simulink model "PTTransmCU"  (Simulink 10.3)
settings: Solver=ode45  StartTime=0.0  StopTime=inf  RelTol=1e-3  EnableMultiTasking=on
libraries: simulink x2, CarMaker4SL x1
(part 5 of 5)

== system PTTransmCU/CarMaker/IPG Vehicle/PowerTrain/TCU Example/TCU GearboxOut/CreateBus TCU GearboxOut0 ==
  In : Inport
  BusCreator : BusCreator  Inputs=7
  Demux : Demux  Outputs=7
      settings: DisplayOption=none
  Out : Outport  VectorParamsAs1DForOutWhenUnconnected=off
  wires:
  Demux/7 -> BusCreator/7  "TCU GearboxOut0 Clutch_dis Pos"
  Demux/6 -> BusCreator/6  "TCU GearboxOut0 Clutch Pos"
  Demux/5 -> BusCreator/5  "TCU GearboxOut0 i_trg"
  Demux/4 -> BusCreator/4  "TCU GearboxOut0 Trq_DriveSrc_trg"
  Demux/3 -> BusCreator/3  "TCU GearboxOut0 set_ParkBrake"
  Demux/2 -> BusCreator/2  "TCU GearboxOut0 GearNoTrg_dis"
  Demux/1 -> BusCreator/1  "TCU GearboxOut0 GearNoTrg"
  BusCreator/1 -> Out/1
  In/1 -> Demux/1

== system PTTransmCU/CarMaker/IPG Vehicle/PowerTrain/TCU Example/TCU GearboxOut/CreateBus TCU GearboxOut1 ==
  In : Inport
  BusCreator : BusCreator  Inputs=7
  Demux : Demux  Outputs=7
      settings: DisplayOption=none
  Out : Outport  VectorParamsAs1DForOutWhenUnconnected=off
  wires:
  Demux/7 -> BusCreator/7  "TCU GearboxOut1 Clutch_dis Pos"
  Demux/6 -> BusCreator/6  "TCU GearboxOut1 Clutch Pos"
  Demux/5 -> BusCreator/5  "TCU GearboxOut1 i_trg"
  Demux/4 -> BusCreator/4  "TCU GearboxOut1 Trq_DriveSrc_trg"
  Demux/3 -> BusCreator/3  "TCU GearboxOut1 set_ParkBrake"
  Demux/2 -> BusCreator/2  "TCU GearboxOut1 GearNoTrg_dis"
  Demux/1 -> BusCreator/1  "TCU GearboxOut1 GearNoTrg"
  BusCreator/1 -> Out/1
  In/1 -> Demux/1

== system PTTransmCU/CarMaker/IPG Vehicle/PowerTrain/TCU Example/TCU GearboxOut/CreateBus TCU GearboxOut10 ==
  In : Inport
  BusCreator : BusCreator  Inputs=7
  Demux : Demux  Outputs=7
      settings: DisplayOption=none
  Out : Outport  VectorParamsAs1DForOutWhenUnconnected=off
  wires:
  Demux/7 -> BusCreator/7  "TCU GearboxOut10 Clutch_dis Pos"
  Demux/6 -> BusCreator/6  "TCU GearboxOut10 Clutch Pos"
  Demux/5 -> BusCreator/5  "TCU GearboxOut10 i_trg"
  Demux/4 -> BusCreator/4  "TCU GearboxOut10 Trq_DriveSrc_trg"
  Demux/3 -> BusCreator/3  "TCU GearboxOut10 set_ParkBrake"
  Demux/2 -> BusCreator/2  "TCU GearboxOut10 GearNoTrg_dis"
  Demux/1 -> BusCreator/1  "TCU GearboxOut10 GearNoTrg"
  BusCreator/1 -> Out/1
  In/1 -> Demux/1

== system PTTransmCU/CarMaker/IPG Vehicle/PowerTrain/TCU Example/TCU GearboxOut/CreateBus TCU GearboxOut11 ==
  In : Inport
  BusCreator : BusCreator  Inputs=7
  Demux : Demux  Outputs=7
      settings: DisplayOption=none
  Out : Outport  VectorParamsAs1DForOutWhenUnconnected=off
  wires:
  Demux/7 -> BusCreator/7  "TCU GearboxOut11 Clutch_dis Pos"
  Demux/6 -> BusCreator/6  "TCU GearboxOut11 Clutch Pos"
  Demux/5 -> BusCreator/5  "TCU GearboxOut11 i_trg"
  Demux/4 -> BusCreator/4  "TCU GearboxOut11 Trq_DriveSrc_trg"
  Demux/3 -> BusCreator/3  "TCU GearboxOut11 set_ParkBrake"
  Demux/2 -> BusCreator/2  "TCU GearboxOut11 GearNoTrg_dis"
  Demux/1 -> BusCreator/1  "TCU GearboxOut11 GearNoTrg"
  BusCreator/1 -> Out/1
  In/1 -> Demux/1

== system PTTransmCU/CarMaker/IPG Vehicle/PowerTrain/TCU Example/TCU GearboxOut/CreateBus TCU GearboxOut2 ==
  In : Inport
  BusCreator : BusCreator  Inputs=7
  Demux : Demux  Outputs=7
      settings: DisplayOption=none
  Out : Outport  VectorParamsAs1DForOutWhenUnconnected=off
  wires:
  Demux/7 -> BusCreator/7  "TCU GearboxOut2 Clutch_dis Pos"
  Demux/6 -> BusCreator/6  "TCU GearboxOut2 Clutch Pos"
  Demux/5 -> BusCreator/5  "TCU GearboxOut2 i_trg"
  Demux/4 -> BusCreator/4  "TCU GearboxOut2 Trq_DriveSrc_trg"
  Demux/3 -> BusCreator/3  "TCU GearboxOut2 set_ParkBrake"
  Demux/2 -> BusCreator/2  "TCU GearboxOut2 GearNoTrg_dis"
  Demux/1 -> BusCreator/1  "TCU GearboxOut2 GearNoTrg"
  BusCreator/1 -> Out/1
  In/1 -> Demux/1

== system PTTransmCU/CarMaker/IPG Vehicle/PowerTrain/TCU Example/TCU GearboxOut/CreateBus TCU GearboxOut3 ==
  In : Inport
  BusCreator : BusCreator  Inputs=7
  Demux : Demux  Outputs=7
      settings: DisplayOption=none
  Out : Outport  VectorParamsAs1DForOutWhenUnconnected=off
  wires:
  Demux/7 -> BusCreator/7  "TCU GearboxOut3 Clutch_dis Pos"
  Demux/6 -> BusCreator/6  "TCU GearboxOut3 Clutch Pos"
  Demux/5 -> BusCreator/5  "TCU GearboxOut3 i_trg"
  Demux/4 -> BusCreator/4  "TCU GearboxOut3 Trq_DriveSrc_trg"
  Demux/3 -> BusCreator/3  "TCU GearboxOut3 set_ParkBrake"
  Demux/2 -> BusCreator/2  "TCU GearboxOut3 GearNoTrg_dis"
  Demux/1 -> BusCreator/1  "TCU GearboxOut3 GearNoTrg"
  BusCreator/1 -> Out/1
  In/1 -> Demux/1

== system PTTransmCU/CarMaker/IPG Vehicle/PowerTrain/TCU Example/TCU GearboxOut/CreateBus TCU GearboxOut4 ==
  In : Inport
  BusCreator : BusCreator  Inputs=7
  Demux : Demux  Outputs=7
      settings: DisplayOption=none
  Out : Outport  VectorParamsAs1DForOutWhenUnconnected=off
  wires:
  Demux/7 -> BusCreator/7  "TCU GearboxOut4 Clutch_dis Pos"
  Demux/6 -> BusCreator/6  "TCU GearboxOut4 Clutch Pos"
  Demux/5 -> BusCreator/5  "TCU GearboxOut4 i_trg"
  Demux/4 -> BusCreator/4  "TCU GearboxOut4 Trq_DriveSrc_trg"
  Demux/3 -> BusCreator/3  "TCU GearboxOut4 set_ParkBrake"
  Demux/2 -> BusCreator/2  "TCU GearboxOut4 GearNoTrg_dis"
  Demux/1 -> BusCreator/1  "TCU GearboxOut4 GearNoTrg"
  BusCreator/1 -> Out/1
  In/1 -> Demux/1

== system PTTransmCU/CarMaker/IPG Vehicle/PowerTrain/TCU Example/TCU GearboxOut/CreateBus TCU GearboxOut5 ==
  In : Inport
  BusCreator : BusCreator  Inputs=7
  Demux : Demux  Outputs=7
      settings: DisplayOption=none
  Out : Outport  VectorParamsAs1DForOutWhenUnconnected=off
  wires:
  Demux/7 -> BusCreator/7  "TCU GearboxOut5 Clutch_dis Pos"
  Demux/6 -> BusCreator/6  "TCU GearboxOut5 Clutch Pos"
  Demux/5 -> BusCreator/5  "TCU GearboxOut5 i_trg"
  Demux/4 -> BusCreator/4  "TCU GearboxOut5 Trq_DriveSrc_trg"
  Demux/3 -> BusCreator/3  "TCU GearboxOut5 set_ParkBrake"
  Demux/2 -> BusCreator/2  "TCU GearboxOut5 GearNoTrg_dis"
  Demux/1 -> BusCreator/1  "TCU GearboxOut5 GearNoTrg"
  BusCreator/1 -> Out/1
  In/1 -> Demux/1

== system PTTransmCU/CarMaker/IPG Vehicle/PowerTrain/TCU Example/TCU GearboxOut/CreateBus TCU GearboxOut6 ==
  In : Inport
  BusCreator : BusCreator  Inputs=7
  Demux : Demux  Outputs=7
      settings: DisplayOption=none
  Out : Outport  VectorParamsAs1DForOutWhenUnconnected=off
  wires:
  Demux/7 -> BusCreator/7  "TCU GearboxOut6 Clutch_dis Pos"
  Demux/6 -> BusCreator/6  "TCU GearboxOut6 Clutch Pos"
  Demux/5 -> BusCreator/5  "TCU GearboxOut6 i_trg"
  Demux/4 -> BusCreator/4  "TCU GearboxOut6 Trq_DriveSrc_trg"
  Demux/3 -> BusCreator/3  "TCU GearboxOut6 set_ParkBrake"
  Demux/2 -> BusCreator/2  "TCU GearboxOut6 GearNoTrg_dis"
  Demux/1 -> BusCreator/1  "TCU GearboxOut6 GearNoTrg"
  BusCreator/1 -> Out/1
  In/1 -> Demux/1

== system PTTransmCU/CarMaker/IPG Vehicle/PowerTrain/TCU Example/TCU GearboxOut/CreateBus TCU GearboxOut7 ==
  In : Inport
  BusCreator : BusCreator  Inputs=7
  Demux : Demux  Outputs=7
      settings: DisplayOption=none
  Out : Outport  VectorParamsAs1DForOutWhenUnconnected=off
  wires:
  Demux/7 -> BusCreator/7  "TCU GearboxOut7 Clutch_dis Pos"
  Demux/6 -> BusCreator/6  "TCU GearboxOut7 Clutch Pos"
  Demux/5 -> BusCreator/5  "TCU GearboxOut7 i_trg"
  Demux/4 -> BusCreator/4  "TCU GearboxOut7 Trq_DriveSrc_trg"
  Demux/3 -> BusCreator/3  "TCU GearboxOut7 set_ParkBrake"
  Demux/2 -> BusCreator/2  "TCU GearboxOut7 GearNoTrg_dis"
  Demux/1 -> BusCreator/1  "TCU GearboxOut7 GearNoTrg"
  BusCreator/1 -> Out/1
  In/1 -> Demux/1

== system PTTransmCU/CarMaker/IPG Vehicle/PowerTrain/TCU Example/TCU GearboxOut/CreateBus TCU GearboxOut8 ==
  In : Inport
  BusCreator : BusCreator  Inputs=7
  Demux : Demux  Outputs=7
      settings: DisplayOption=none
  Out : Outport  VectorParamsAs1DForOutWhenUnconnected=off
  wires:
  Demux/7 -> BusCreator/7  "TCU GearboxOut8 Clutch_dis Pos"
  Demux/6 -> BusCreator/6  "TCU GearboxOut8 Clutch Pos"
  Demux/5 -> BusCreator/5  "TCU GearboxOut8 i_trg"
  Demux/4 -> BusCreator/4  "TCU GearboxOut8 Trq_DriveSrc_trg"
  Demux/3 -> BusCreator/3  "TCU GearboxOut8 set_ParkBrake"
  Demux/2 -> BusCreator/2  "TCU GearboxOut8 GearNoTrg_dis"
  Demux/1 -> BusCreator/1  "TCU GearboxOut8 GearNoTrg"
  BusCreator/1 -> Out/1
  In/1 -> Demux/1

== system PTTransmCU/CarMaker/IPG Vehicle/PowerTrain/TCU Example/TCU GearboxOut/CreateBus TCU GearboxOut9 ==
  In : Inport
  BusCreator : BusCreator  Inputs=7
  Demux : Demux  Outputs=7
      settings: DisplayOption=none
  Out : Outport  VectorParamsAs1DForOutWhenUnconnected=off
  wires:
  Demux/7 -> BusCreator/7  "TCU GearboxOut9 Clutch_dis Pos"
  Demux/6 -> BusCreator/6  "TCU GearboxOut9 Clutch Pos"
  Demux/5 -> BusCreator/5  "TCU GearboxOut9 i_trg"
  Demux/4 -> BusCreator/4  "TCU GearboxOut9 Trq_DriveSrc_trg"
  Demux/3 -> BusCreator/3  "TCU GearboxOut9 set_ParkBrake"
  Demux/2 -> BusCreator/2  "TCU GearboxOut9 GearNoTrg_dis"
  Demux/1 -> BusCreator/1  "TCU GearboxOut9 GearNoTrg"
  BusCreator/1 -> Out/1
  In/1 -> Demux/1

== system PTTransmCU/CarMaker/IPG Vehicle/PowerTrain/TCU Example/TCU Example/Calculate GearNoTrg/Backwards ==
  Action Port : ActionPort  ActionPortLabel=case: { }
  Constant : Constant  Value=-1
  GearNoTrg : Outport  InitialOutput=-1  VectorParamsAs1DForOutWhenUnconnected=off
  wires:
  Constant/1 -> GearNoTrg/1

== system PTTransmCU/CarMaker/IPG Vehicle/PowerTrain/TCU Example/TCU Example/Calculate GearNoTrg/Driving ==
  GearNo : Inport
  Upper Limit : Inport  Port=2
  Lower Limit : Inport  Port=3
  rotvRef : Inport  Port=4
  nFGears : Inport  Port=5
  GearNoTrg_last : Inport  Port=6
  Action Port : ActionPort  ActionPortLabel=case: { }
  Bias : Bias  Bias=-1
  Bias1 : Bias  Bias=1
  Constant : Constant
  Constant1 : Constant
  Subsystem : Subsystem
  Subsystem1 : Subsystem
  Switch : Switch  Criteria=u2 ~= 0
  Switch1 : Switch  Criteria=u2 ~= 0
  Switch2 : Switch  Criteria=u2 ~= 0
  Switch3 : Switch  Criteria=u2 > Threshold
  GearNoTrg : Outport  InitialOutput=1  VectorParamsAs1DForOutWhenUnconnected=off
  wires:
  Constant1/1 -> Switch3/3
  GearNoTrg_last/1 -> Switch3/1, Switch3/2
  Switch3/1 -> Switch1/3
  Lower Limit/1 -> Subsystem1/3(Lower Limit)
  Subsystem1/1(Out1) -> Switch1/2
  nFGears/1 -> Subsystem/4(nFGears)
  Upper Limit/1 -> Subsystem/3(Upper Limit)
  Subsystem/1(Out1) -> Switch2/2
  Bias1/1 -> Switch2/1
  Bias/1 -> Switch1/1
  Switch1/1 -> Switch2/3
  Switch2/1 -> Switch/1
  rotvRef/1 -> Subsystem1/1(rotvRef), Subsystem/1(rotvRef)
  Switch/1 -> GearNoTrg/1
  Constant/1 -> Switch/3
  GearNo/1 -> Switch/2, Subsystem1/2(GearNo), Subsystem/2(GearNo), Bias1/1, Bias/1

== system PTTransmCU/CarMaker/IPG Vehicle/PowerTrain/TCU Example/TCU Example/Calculate GearNoTrg/else ==
  Action Port : ActionPort  ActionPortLabel=default: { }
  Constant : Constant  Value=0
  GearNoTrg : Outport  InitialOutput=0  VectorParamsAs1DForOutWhenUnconnected=off
  wires:
  Constant/1 -> GearNoTrg/1

== system PTTransmCU/CarMaker/IPG Vehicle/PowerTrain/TCU Example/TCU Example/Calculate GearNoTrg/Driving/Subsystem ==
  rotvRef : Inport
  GearNo : Inport  Port=2
  Upper Limit : Inport  Port=3
  nFGears : Inport  Port=4
  Logical Operator : Logic  AllPortsSameDT=off  OutDataTypeStr=boolean
  Relational Operator1 : RelationalOperator  OutDataTypeStr=boolean  RndMeth=Nearest
  Relational Operator2 : RelationalOperator  Operator=<  OutDataTypeStr=boolean  RndMeth=Nearest
  Out1 : Outport  VectorParamsAs1DForOutWhenUnconnected=off
  wires:
  Relational Operator2/1 -> Logical Operator/2
  nFGears/1 -> Relational Operator2/2
  GearNo/1 -> Relational Operator2/1
  Logical Operator/1 -> Out1/1
  Relational Operator1/1 -> Logical Operator/1
  Upper Limit/1 -> Relational Operator1/2
  rotvRef/1 -> Relational Operator1/1

== system PTTransmCU/CarMaker/IPG Vehicle/PowerTrain/TCU Example/TCU Example/Calculate GearNoTrg/Driving/Subsystem1 ==
  rotvRef : Inport
  GearNo : Inport  Port=2
  Lower Limit : Inport  Port=3
  Constant : Constant
  Logical Operator : Logic  AllPortsSameDT=off  OutDataTypeStr=boolean
  Relational Operator1 : RelationalOperator  Operator=<=  OutDataTypeStr=boolean  RndMeth=Nearest
  Relational Operator2 : RelationalOperator  Operator=>  OutDataTypeStr=boolean  RndMeth=Nearest
  Out1 : Outport  VectorParamsAs1DForOutWhenUnconnected=off
  wires:
  Relational Operator2/1 -> Logical Operator/2
  Constant/1 -> Relational Operator2/2
  GearNo/1 -> Relational Operator2/1
  Logical Operator/1 -> Out1/1
  Relational Operator1/1 -> Logical Operator/1
  Lower Limit/1 -> Relational Operator1/2
  rotvRef/1 -> Relational Operator1/1
